simulink model "Grap"  (R2015a)
settings: Solver=ode45  StartTime=0.0  StopTime=10.0  RelTol=1e-3
undefined symbols (not defined in the file or in its folder): Eff, gear, gear_ratio, Required_power, Rtyre
settings Model: Creator=DELL  LastModifiedBy=DELL

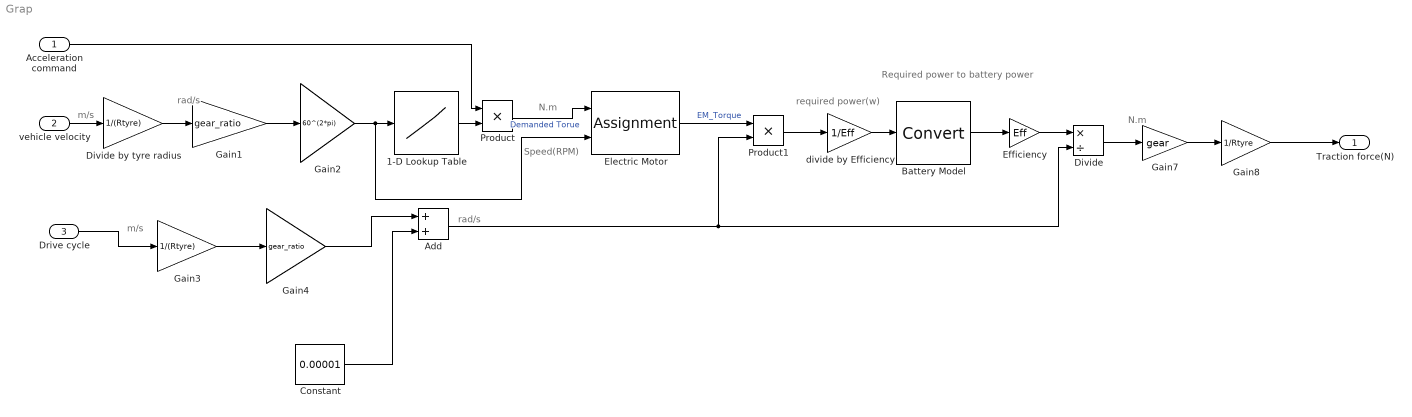
== system Grap ==
  note: m/s
  note: Required power to battery power
  note: m/s
  note: rad/s
  note: N.m
  note: required
      | power(w)
  note: N.m
  note: rad/s
  note: Speed(RPM)
  "Acceleration command " : Inport
  vehicle velocity : Inport  Port=2
  Drive cycle : Inport  Port=3
  1-D Lookup Table : Lookup_n-D  NumberOfTableDimensions=1  BreakpointsForDimension1=[-5:5]  Table=tanh([-5:5])  InternalRulePriority=Speed  RndMeth=Simplest  InputSameDT=on
  Add : Sum
  Battery Model : DataTypeConversion  OutMin=Required_power
  Constant : Constant  Value=0.00001
  Divide : Product  Inputs=*/
  Divide by tyre radius : Gain  Gain=1/(Rtyre)
  Efficiency : Gain  Gain=Eff
  "Electric Motor " : Assignment  DiagnosticForDimensions=Warning
  Gain1 : Gain  Gain=gear_ratio
  Gain2 : Gain  Gain=60^(2*pi)
  Gain3 : Gain  Gain=1/(Rtyre)
  Gain4 : Gain  Gain=gear_ratio
  Gain7 : Gain  Gain=gear
  Gain8 : Gain  Gain=1/Rtyre
  Product : Product
  Product1 : Product
  divide by Efficiency : Gain  Gain=1/Eff
  Traction force(N) : Outport
  wires:
  Divide by tyre radius/1 -> Gain1/1
  Gain1/1 -> Gain2/1
  vehicle velocity/1 -> Divide by tyre radius/1
  1-D Lookup Table/1 -> Product/2
  "Acceleration command "/1 -> Product/1
  "Electric Motor "/1 -> Product1/1  "EM_Torque"
  Drive cycle/1 -> Gain3/1
  Gain3/1 -> Gain4/1
  Gain4/1 -> Add/1
  Constant/1 -> Add/2
  Product1/1 -> divide by Efficiency/1
  divide by Efficiency/1 -> Battery Model/1
  Battery Model/1 -> Efficiency/1
  Efficiency/1 -> Divide/1
  Add/1 -> Divide/2, Product1/2
  Divide/1 -> Gain7/1
  Gain7/1 -> Gain8/1
  Gain8/1 -> Traction force(N)/1
  Product/1 -> "Electric Motor "/1  "Demanded Torue"
  Gain2/1 -> "Electric Motor "/2, 1-D Lookup Table/1
